simulink model "power_13NodeTestFeeder_4VSC_PV_DEG_symmtrc_loads_"  (R2024b)
settings: Solver=ode15s  StartTime=0.0  StopTime=5  FixedStep=1e-6  MaxStep=1e-4  RelTol=1e-6  AbsTol=1e-8  EnableMultiTasking=on
PreLoadFcn:
  | %power_13NodeTestFeeder_init;
values from neighbouring files (symbols this model uses):
  a = 1.3    [init_para_with_symmtrc_loads.m]
  Cdc = 278e-3    (= 0.278)    [init_para_with_symmtrc_loads.m]
  fg = 60    [a01_scan_VSC_13_feeder.m]    (also in init_para_with_symmtrc_loads.m)
  Gn = 1000    [init_para_with_symmtrc_loads.m]
  H = 8    [init_para_with_symmtrc_loads.m]
  Ipv_n = Isc_n*(Rp+Rs)/Rp    (= 8.21426513558)    [init_para_with_symmtrc_loads.m]
  Isc_n = 8.21    [init_para_with_symmtrc_loads.m]
  k = 1.3806503e-23    [init_para_with_symmtrc_loads.m]    (also in ypm_plot_compare_ana_meas.m = 2)
  Kdroop = Sn/(Rdroop*60)    (= 4166666.66667)    [init_para_with_symmtrc_loads.m]
  KI = 0.0032    [init_para_with_symmtrc_loads.m]
  Ki_C = Rc/tau_C    (= 0.768)    [init_para_with_symmtrc_loads.m]
  Ki_DC = omega_DC^2*Cdc    [init_para_with_symmtrc_loads.m]
  ki_dvpp = kp_dvpp/Ti_dvpp    [init_para_with_symmtrc_loads.m]
  Ki_P = 1/(Ki_pq*tau_P)    [init_para_with_symmtrc_loads.m]
  Ki_PLL = Kp_PLL/tau_PLL    [init_para_with_symmtrc_loads.m]
  Kp_C = Lc/tau_C    (= 0.020372)    [init_para_with_symmtrc_loads.m]
  Kp_DC = 2*xi_DC*omega_DC*Cdc    [init_para_with_symmtrc_loads.m]
  kp_dvpp = -(2*Kdcgain)^-1    [init_para_with_symmtrc_loads.m]
  Kp_P = tau_C/(Ki_pq*tau_P)    [init_para_with_symmtrc_loads.m]
  Kp_PLL = xi_PLL*2*omega_PLL/Vp    [init_para_with_symmtrc_loads.m]
  KV = -0.123    [init_para_with_symmtrc_loads.m]
  kv_Vp = [ 1.021 1.042 1.0174]    [init_para_with_symmtrc_loads.m]
  KVmp = Vmp_n/Voc_n    (= 0.799392097264)    [init_para_with_symmtrc_loads.m]
  Lc = 20.372e-6    (= 2.0372e-05)    [init_para_with_symmtrc_loads.m]
  Lg = Xg /(2*pi*fg)    [init_para_with_symmtrc_loads.m]
  Np = 345    [init_para_with_symmtrc_loads.m]
  Ns = 45    [init_para_with_symmtrc_loads.m]
  Ns_cell = 54    [init_para_with_symmtrc_loads.m]
  p_jump_time = 5    [init_para_with_symmtrc_loads.m]
  p_jump_value = 2*-1e6    (= -2000000)    [init_para_with_symmtrc_loads.m]
  phi_vec = phi_vec_deg/180*pi    [init_para_with_symmtrc_loads.m]
  ppv_nom = 4.9687e+05    (= 496870)    [init_para_with_symmtrc_loads.m]
  q = 1.6021764e-19    [init_para_with_symmtrc_loads.m]
  Rc = 0.768e-3    (= 0.000768)    [init_para_with_symmtrc_loads.m]
  Rg = (U_rms^2 / S_sc) / (sqrt(1 + XoverR^2))    [init_para_with_symmtrc_loads.m]
  Rp = 425.405    [init_para_with_symmtrc_loads.m]
  Rs = 0.221    [init_para_with_symmtrc_loads.m]
  S_base_all = 1    [init_para_with_symmtrc_loads.m]
  Sn = 15e6    (= 15000000)    [init_para_with_symmtrc_loads.m]
  tau_PLL = 2*xi_PLL/omega_PLL    [init_para_with_symmtrc_loads.m]
  Tn = 25    [init_para_with_symmtrc_loads.m]
  Ts = T_ctrl/n_ctrl    [a01_scan_VSC_13_feeder.m]    (also in init_para_with_symmtrc_loads.m = 5e-05)
  U_rms = 4160    [init_para_with_symmtrc_loads.m]
  Vdc = 1200    [init_para_with_symmtrc_loads.m]
  Voc_n = 32.9    [init_para_with_symmtrc_loads.m]
  Vp = sqrt(2)*480/sqrt(3)    [a01_scan_VSC_13_feeder.m]    (also in init_para_with_symmtrc_loads.m = Ug*sqrt(2)/sqrt(3))
undefined symbols (not defined in the file or in its folder): j, Newton, para_grid, para_PVgeno, Raphson
libraries: spsabctoAlphaBetaZeroLib x141, spsPower3phInstantaneousLib x70, spsSeriesRLCBranchLib x44, spsThreePhaseVIMeasurementLib x27, slpidlib x24, spsThreePhaseSeriesRLCLoadLib x15, spsControlledVoltageSourceLib x15, spsMeanLib x9, spsCurrentMeasurementLib x8, spsControlledCurrentSourceLib x8, cstblocks x8, spsGroundLib x5
(part 6 of 10)

== system power_13NodeTestFeeder_4VSC_PV_DEG_symmtrc_loads_/V I P Q Measurements EMT_without scopes_with_logsout/PQ_12 ==
  U : Inport
  I : Inport  Port=2
  Complex to Magnitude-Angle1 : ComplexToMagnitudeAngle
  Complex to Magnitude-Angle2 : ComplexToMagnitudeAngle
  Complex to Real-Imag : ComplexToRealImag
  Demux : Demux  Outputs=3
  Demux1 : Demux  Outputs=3
  Gain : Gain  Gain=1/S_base_all
  Gain1 : Gain  Gain=j
  Mux : Mux  Inputs=2
  "Power (3ph, Instantaneous)1" : spsPower3phInstantaneousLib/Power (3ph, Instantaneous)
  Real-Imag to Complex : RealImagToComplex
  Real-Imag to Complex1 : RealImagToComplex
  Sum : Sum  Inputs=|++
  Terminator{1,3,5..8} (6 alike) : Terminator
  Transfer Fcn{1..4} (4 alike) : TransferFcn  Denominator=[1e-3 1]
  abc to Alpha-Beta-Zero : spsabctoAlphaBetaZeroLib/abc to Alpha-Beta-Zero
  abc to Alpha-Beta-Zero1 : spsabctoAlphaBetaZeroLib/abc to Alpha-Beta-Zero
  PQ : Outport
  wires:
  I/1 -> abc to Alpha-Beta-Zero1/1, "Power (3ph, Instantaneous)1"/2
  Gain1/1 -> Sum/2
  Complex to Real-Imag/1 -> Mux/1
  Complex to Real-Imag/2 -> Mux/2
  Mux/1 -> PQ/1
  "Power (3ph, Instantaneous)1"/2 -> Transfer Fcn2/1
  "Power (3ph, Instantaneous)1"/1 -> Transfer Fcn1/1
  Sum/1 -> Gain/1
  Gain/1 -> Complex to Real-Imag/1
  U/1 -> abc to Alpha-Beta-Zero/1, "Power (3ph, Instantaneous)1"/1
  abc to Alpha-Beta-Zero/1 -> Demux/1
  Demux/1 -> Real-Imag to Complex/1
  Demux/2 -> Real-Imag to Complex/2
  Real-Imag to Complex/1 -> Complex to Magnitude-Angle2/1
  Complex to Magnitude-Angle2/1 -> Transfer Fcn3/1
  Complex to Magnitude-Angle2/2 -> Terminator3/1
  Complex to Magnitude-Angle1/1 -> Transfer Fcn4/1
  Real-Imag to Complex1/1 -> Complex to Magnitude-Angle1/1
  Demux1/2 -> Real-Imag to Complex1/2
  Demux1/1 -> Real-Imag to Complex1/1
  abc to Alpha-Beta-Zero1/1 -> Demux1/1
  Transfer Fcn1/1 -> Sum/1  "p"
  Transfer Fcn2/1 -> Gain1/1  "p"
  Transfer Fcn3/1 -> Terminator6/1  "u_betrag"
  Transfer Fcn4/1 -> Terminator5/1  "i_betrag"
  Demux1/3 -> Terminator7/1
  Demux/3 -> Terminator8/1
  Complex to Magnitude-Angle1/2 -> Terminator1/1

== system power_13NodeTestFeeder_4VSC_PV_DEG_symmtrc_loads_/V I P Q Measurements EMT_without scopes_with_logsout/PQ_13 ==
  U : Inport
  I : Inport  Port=2
  Complex to Magnitude-Angle1 : ComplexToMagnitudeAngle
  Complex to Magnitude-Angle2 : ComplexToMagnitudeAngle
  Complex to Real-Imag : ComplexToRealImag
  Demux : Demux  Outputs=3
  Demux1 : Demux  Outputs=3
  Gain : Gain  Gain=1/S_base_all
  Gain1 : Gain  Gain=j
  Mux : Mux  Inputs=2
  "Power (3ph, Instantaneous)1" : spsPower3phInstantaneousLib/Power (3ph, Instantaneous)
  Real-Imag to Complex : RealImagToComplex
  Real-Imag to Complex1 : RealImagToComplex
  Sum : Sum  Inputs=|++
  Terminator{1,3,5..8} (6 alike) : Terminator
  Transfer Fcn{1..4} (4 alike) : TransferFcn  Denominator=[1e-3 1]
  abc to Alpha-Beta-Zero : spsabctoAlphaBetaZeroLib/abc to Alpha-Beta-Zero
  abc to Alpha-Beta-Zero1 : spsabctoAlphaBetaZeroLib/abc to Alpha-Beta-Zero
  PQ : Outport
  wires:
  I/1 -> abc to Alpha-Beta-Zero1/1, "Power (3ph, Instantaneous)1"/2
  Gain1/1 -> Sum/2
  Complex to Real-Imag/1 -> Mux/1
  Complex to Real-Imag/2 -> Mux/2
  Mux/1 -> PQ/1
  "Power (3ph, Instantaneous)1"/2 -> Transfer Fcn2/1
  "Power (3ph, Instantaneous)1"/1 -> Transfer Fcn1/1
  Sum/1 -> Gain/1
  Gain/1 -> Complex to Real-Imag/1
  U/1 -> abc to Alpha-Beta-Zero/1, "Power (3ph, Instantaneous)1"/1
  abc to Alpha-Beta-Zero/1 -> Demux/1
  Demux/1 -> Real-Imag to Complex/1
  Demux/2 -> Real-Imag to Complex/2
  Real-Imag to Complex/1 -> Complex to Magnitude-Angle2/1
  Complex to Magnitude-Angle2/1 -> Transfer Fcn3/1
  Complex to Magnitude-Angle2/2 -> Terminator3/1
  Complex to Magnitude-Angle1/1 -> Transfer Fcn4/1
  Real-Imag to Complex1/1 -> Complex to Magnitude-Angle1/1
  Demux1/2 -> Real-Imag to Complex1/2
  Demux1/1 -> Real-Imag to Complex1/1
  abc to Alpha-Beta-Zero1/1 -> Demux1/1
  Transfer Fcn1/1 -> Sum/1  "p"
  Transfer Fcn2/1 -> Gain1/1  "p"
  Transfer Fcn3/1 -> Terminator6/1  "u_betrag"
  Transfer Fcn4/1 -> Terminator5/1  "i_betrag"
  Demux1/3 -> Terminator7/1
  Demux/3 -> Terminator8/1
  Complex to Magnitude-Angle1/2 -> Terminator1/1

== system power_13NodeTestFeeder_4VSC_PV_DEG_symmtrc_loads_/V I P Q Measurements EMT_without scopes_with_logsout/PQ_14 ==
  U : Inport
  I : Inport  Port=2
  Complex to Magnitude-Angle1 : ComplexToMagnitudeAngle
  Complex to Magnitude-Angle2 : ComplexToMagnitudeAngle
  Complex to Real-Imag : ComplexToRealImag
  Demux : Demux  Outputs=3
  Demux1 : Demux  Outputs=3
  Gain : Gain  Gain=1/S_base_all
  Gain1 : Gain  Gain=j
  Mux : Mux  Inputs=2
  "Power (3ph, Instantaneous)1" : spsPower3phInstantaneousLib/Power (3ph, Instantaneous)
  Real-Imag to Complex : RealImagToComplex
  Real-Imag to Complex1 : RealImagToComplex
  Sum : Sum  Inputs=|++
  Terminator{1,3,5..8} (6 alike) : Terminator
  Transfer Fcn{1..4} (4 alike) : TransferFcn  Denominator=[1e-3 1]
  abc to Alpha-Beta-Zero : spsabctoAlphaBetaZeroLib/abc to Alpha-Beta-Zero
  abc to Alpha-Beta-Zero1 : spsabctoAlphaBetaZeroLib/abc to Alpha-Beta-Zero
  PQ : Outport
  wires:
  I/1 -> abc to Alpha-Beta-Zero1/1, "Power (3ph, Instantaneous)1"/2
  Gain1/1 -> Sum/2
  Complex to Real-Imag/1 -> Mux/1
  Complex to Real-Imag/2 -> Mux/2
  Mux/1 -> PQ/1
  "Power (3ph, Instantaneous)1"/2 -> Transfer Fcn2/1
  "Power (3ph, Instantaneous)1"/1 -> Transfer Fcn1/1
  Sum/1 -> Gain/1
  Gain/1 -> Complex to Real-Imag/1
  U/1 -> abc to Alpha-Beta-Zero/1, "Power (3ph, Instantaneous)1"/1
  abc to Alpha-Beta-Zero/1 -> Demux/1
  Demux/1 -> Real-Imag to Complex/1
  Demux/2 -> Real-Imag to Complex/2
  Real-Imag to Complex/1 -> Complex to Magnitude-Angle2/1
  Complex to Magnitude-Angle2/1 -> Transfer Fcn3/1
  Complex to Magnitude-Angle2/2 -> Terminator3/1
  Complex to Magnitude-Angle1/1 -> Transfer Fcn4/1
  Real-Imag to Complex1/1 -> Complex to Magnitude-Angle1/1
  Demux1/2 -> Real-Imag to Complex1/2
  Demux1/1 -> Real-Imag to Complex1/1
  abc to Alpha-Beta-Zero1/1 -> Demux1/1
  Transfer Fcn1/1 -> Sum/1  "p"
  Transfer Fcn2/1 -> Gain1/1  "p"
  Transfer Fcn3/1 -> Terminator6/1  "u_betrag"
  Transfer Fcn4/1 -> Terminator5/1  "i_betrag"
  Demux1/3 -> Terminator7/1
  Demux/3 -> Terminator8/1
  Complex to Magnitude-Angle1/2 -> Terminator1/1

== system power_13NodeTestFeeder_4VSC_PV_DEG_symmtrc_loads_/V I P Q Measurements EMT_without scopes_with_logsout/PQ_15 ==
  U : Inport
  I : Inport  Port=2
  Complex to Magnitude-Angle1 : ComplexToMagnitudeAngle
  Complex to Magnitude-Angle2 : ComplexToMagnitudeAngle
  Complex to Real-Imag : ComplexToRealImag
  Demux : Demux  Outputs=3
  Demux1 : Demux  Outputs=3
  Gain : Gain  Gain=1/S_base_all
  Gain1 : Gain  Gain=j
  Mux : Mux  Inputs=2
  "Power (3ph, Instantaneous)1" : spsPower3phInstantaneousLib/Power (3ph, Instantaneous)
  Real-Imag to Complex : RealImagToComplex
  Real-Imag to Complex1 : RealImagToComplex
  Sum : Sum  Inputs=|++
  Terminator{1,3,5..8} (6 alike) : Terminator
  Transfer Fcn{1..4} (4 alike) : TransferFcn  Denominator=[1e-3 1]
  abc to Alpha-Beta-Zero : spsabctoAlphaBetaZeroLib/abc to Alpha-Beta-Zero
  abc to Alpha-Beta-Zero1 : spsabctoAlphaBetaZeroLib/abc to Alpha-Beta-Zero
  PQ : Outport
  wires:
  I/1 -> abc to Alpha-Beta-Zero1/1, "Power (3ph, Instantaneous)1"/2
  Gain1/1 -> Sum/2
  Complex to Real-Imag/1 -> Mux/1
  Complex to Real-Imag/2 -> Mux/2
  Mux/1 -> PQ/1
  "Power (3ph, Instantaneous)1"/2 -> Transfer Fcn2/1
  "Power (3ph, Instantaneous)1"/1 -> Transfer Fcn1/1
  Sum/1 -> Gain/1
  Gain/1 -> Complex to Real-Imag/1
  U/1 -> abc to Alpha-Beta-Zero/1, "Power (3ph, Instantaneous)1"/1
  abc to Alpha-Beta-Zero/1 -> Demux/1
  Demux/1 -> Real-Imag to Complex/1
  Demux/2 -> Real-Imag to Complex/2
  Real-Imag to Complex/1 -> Complex to Magnitude-Angle2/1
  Complex to Magnitude-Angle2/1 -> Transfer Fcn3/1
  Complex to Magnitude-Angle2/2 -> Terminator3/1
  Complex to Magnitude-Angle1/1 -> Transfer Fcn4/1
  Real-Imag to Complex1/1 -> Complex to Magnitude-Angle1/1
  Demux1/2 -> Real-Imag to Complex1/2
  Demux1/1 -> Real-Imag to Complex1/1
  abc to Alpha-Beta-Zero1/1 -> Demux1/1
  Transfer Fcn1/1 -> Sum/1  "p"
  Transfer Fcn2/1 -> Gain1/1  "p"
  Transfer Fcn3/1 -> Terminator6/1  "u_betrag"
  Transfer Fcn4/1 -> Terminator5/1  "i_betrag"
  Demux1/3 -> Terminator7/1
  Demux/3 -> Terminator8/1
  Complex to Magnitude-Angle1/2 -> Terminator1/1

== system power_13NodeTestFeeder_4VSC_PV_DEG_symmtrc_loads_/V I P Q Measurements EMT_without scopes_with_logsout/PQ_16 ==
  U : Inport
  I : Inport  Port=2
  Complex to Magnitude-Angle1 : ComplexToMagnitudeAngle
  Complex to Magnitude-Angle2 : ComplexToMagnitudeAngle
  Complex to Real-Imag : ComplexToRealImag
  Demux : Demux  Outputs=3
  Demux1 : Demux  Outputs=3
  Gain : Gain  Gain=1/S_base_all
  Gain1 : Gain  Gain=j
  Mux : Mux  Inputs=2
  "Power (3ph, Instantaneous)1" : spsPower3phInstantaneousLib/Power (3ph, Instantaneous)
  Real-Imag to Complex : RealImagToComplex
  Real-Imag to Complex1 : RealImagToComplex
  Sum : Sum  Inputs=|++
  Terminator{1,3,5..8} (6 alike) : Terminator
  Transfer Fcn{1..4} (4 alike) : TransferFcn  Denominator=[1e-3 1]
  abc to Alpha-Beta-Zero : spsabctoAlphaBetaZeroLib/abc to Alpha-Beta-Zero
  abc to Alpha-Beta-Zero1 : spsabctoAlphaBetaZeroLib/abc to Alpha-Beta-Zero
  PQ : Outport
  wires:
  I/1 -> abc to Alpha-Beta-Zero1/1, "Power (3ph, Instantaneous)1"/2
  Gain1/1 -> Sum/2
  Complex to Real-Imag/1 -> Mux/1
  Complex to Real-Imag/2 -> Mux/2
  Mux/1 -> PQ/1
  "Power (3ph, Instantaneous)1"/2 -> Transfer Fcn2/1
  "Power (3ph, Instantaneous)1"/1 -> Transfer Fcn1/1
  Sum/1 -> Gain/1
  Gain/1 -> Complex to Real-Imag/1
  U/1 -> abc to Alpha-Beta-Zero/1, "Power (3ph, Instantaneous)1"/1
  abc to Alpha-Beta-Zero/1 -> Demux/1
  Demux/1 -> Real-Imag to Complex/1
  Demux/2 -> Real-Imag to Complex/2
  Real-Imag to Complex/1 -> Complex to Magnitude-Angle2/1
  Complex to Magnitude-Angle2/1 -> Transfer Fcn3/1
  Complex to Magnitude-Angle2/2 -> Terminator3/1
  Complex to Magnitude-Angle1/1 -> Transfer Fcn4/1
  Real-Imag to Complex1/1 -> Complex to Magnitude-Angle1/1
  Demux1/2 -> Real-Imag to Complex1/2
  Demux1/1 -> Real-Imag to Complex1/1
  abc to Alpha-Beta-Zero1/1 -> Demux1/1
  Transfer Fcn1/1 -> Sum/1  "p"
  Transfer Fcn2/1 -> Gain1/1  "p"
  Transfer Fcn3/1 -> Terminator6/1  "u_betrag"
  Transfer Fcn4/1 -> Terminator5/1  "i_betrag"
  Demux1/3 -> Terminator7/1
  Demux/3 -> Terminator8/1
  Complex to Magnitude-Angle1/2 -> Terminator1/1

== system power_13NodeTestFeeder_4VSC_PV_DEG_symmtrc_loads_/V I P Q Measurements EMT_without scopes_with_logsout/PQ_17 ==
  U : Inport
  I : Inport  Port=2
  Complex to Magnitude-Angle1 : ComplexToMagnitudeAngle
  Complex to Magnitude-Angle2 : ComplexToMagnitudeAngle
  Complex to Real-Imag : ComplexToRealImag
  Demux : Demux  Outputs=3
  Demux1 : Demux  Outputs=3
  Gain : Gain  Gain=1/S_base_all
  Gain1 : Gain  Gain=j
  Mux : Mux  Inputs=2
  "Power (3ph, Instantaneous)1" : spsPower3phInstantaneousLib/Power (3ph, Instantaneous)
  Real-Imag to Complex : RealImagToComplex
  Real-Imag to Complex1 : RealImagToComplex
  Sum : Sum  Inputs=|++
  Terminator{1,3,5..8} (6 alike) : Terminator
  Transfer Fcn{1..4} (4 alike) : TransferFcn  Denominator=[1e-3 1]
  abc to Alpha-Beta-Zero : spsabctoAlphaBetaZeroLib/abc to Alpha-Beta-Zero
  abc to Alpha-Beta-Zero1 : spsabctoAlphaBetaZeroLib/abc to Alpha-Beta-Zero
  PQ : Outport
  wires:
  I/1 -> abc to Alpha-Beta-Zero1/1, "Power (3ph, Instantaneous)1"/2
  Gain1/1 -> Sum/2
  Complex to Real-Imag/1 -> Mux/1
  Complex to Real-Imag/2 -> Mux/2
  Mux/1 -> PQ/1
  "Power (3ph, Instantaneous)1"/2 -> Transfer Fcn2/1
  "Power (3ph, Instantaneous)1"/1 -> Transfer Fcn1/1
  Sum/1 -> Gain/1
  Gain/1 -> Complex to Real-Imag/1
  U/1 -> abc to Alpha-Beta-Zero/1, "Power (3ph, Instantaneous)1"/1
  abc to Alpha-Beta-Zero/1 -> Demux/1
  Demux/1 -> Real-Imag to Complex/1
  Demux/2 -> Real-Imag to Complex/2
  Real-Imag to Complex/1 -> Complex to Magnitude-Angle2/1
  Complex to Magnitude-Angle2/1 -> Transfer Fcn3/1
  Complex to Magnitude-Angle2/2 -> Terminator3/1
  Complex to Magnitude-Angle1/1 -> Transfer Fcn4/1
  Real-Imag to Complex1/1 -> Complex to Magnitude-Angle1/1
  Demux1/2 -> Real-Imag to Complex1/2
  Demux1/1 -> Real-Imag to Complex1/1
  abc to Alpha-Beta-Zero1/1 -> Demux1/1
  Transfer Fcn1/1 -> Sum/1  "p"
  Transfer Fcn2/1 -> Gain1/1  "p"
  Transfer Fcn3/1 -> Terminator6/1  "u_betrag"
  Transfer Fcn4/1 -> Terminator5/1  "i_betrag"
  Demux1/3 -> Terminator7/1
  Demux/3 -> Terminator8/1
  Complex to Magnitude-Angle1/2 -> Terminator1/1

== system power_13NodeTestFeeder_4VSC_PV_DEG_symmtrc_loads_/V I P Q Measurements EMT_without scopes_with_logsout/PQ_18 ==
  U : Inport
  I : Inport  Port=2
  Complex to Magnitude-Angle1 : ComplexToMagnitudeAngle
  Complex to Magnitude-Angle2 : ComplexToMagnitudeAngle
  Complex to Real-Imag : ComplexToRealImag
  Demux : Demux  Outputs=3
  Demux1 : Demux  Outputs=3
  Gain : Gain  Gain=1/S_base_all
  Gain1 : Gain  Gain=j
  Mux : Mux  Inputs=2
  "Power (3ph, Instantaneous)1" : spsPower3phInstantaneousLib/Power (3ph, Instantaneous)
  Real-Imag to Complex : RealImagToComplex
  Real-Imag to Complex1 : RealImagToComplex
  Sum : Sum  Inputs=|++
  Terminator{1,3,5..8} (6 alike) : Terminator
  Transfer Fcn{1..4} (4 alike) : TransferFcn  Denominator=[1e-3 1]
  abc to Alpha-Beta-Zero : spsabctoAlphaBetaZeroLib/abc to Alpha-Beta-Zero
  abc to Alpha-Beta-Zero1 : spsabctoAlphaBetaZeroLib/abc to Alpha-Beta-Zero
  PQ : Outport
  wires:
  I/1 -> abc to Alpha-Beta-Zero1/1, "Power (3ph, Instantaneous)1"/2
  Gain1/1 -> Sum/2
  Complex to Real-Imag/1 -> Mux/1
  Complex to Real-Imag/2 -> Mux/2
  Mux/1 -> PQ/1
  "Power (3ph, Instantaneous)1"/2 -> Transfer Fcn2/1
  "Power (3ph, Instantaneous)1"/1 -> Transfer Fcn1/1
  Sum/1 -> Gain/1
  Gain/1 -> Complex to Real-Imag/1
  U/1 -> abc to Alpha-Beta-Zero/1, "Power (3ph, Instantaneous)1"/1
  abc to Alpha-Beta-Zero/1 -> Demux/1
  Demux/1 -> Real-Imag to Complex/1
  Demux/2 -> Real-Imag to Complex/2
  Real-Imag to Complex/1 -> Complex to Magnitude-Angle2/1
  Complex to Magnitude-Angle2/1 -> Transfer Fcn3/1
  Complex to Magnitude-Angle2/2 -> Terminator3/1
  Complex to Magnitude-Angle1/1 -> Transfer Fcn4/1
  Real-Imag to Complex1/1 -> Complex to Magnitude-Angle1/1
  Demux1/2 -> Real-Imag to Complex1/2
  Demux1/1 -> Real-Imag to Complex1/1
  abc to Alpha-Beta-Zero1/1 -> Demux1/1
  Transfer Fcn1/1 -> Sum/1  "p"
  Transfer Fcn2/1 -> Gain1/1  "p"
  Transfer Fcn3/1 -> Terminator6/1  "u_betrag"
  Transfer Fcn4/1 -> Terminator5/1  "i_betrag"
  Demux1/3 -> Terminator7/1
  Demux/3 -> Terminator8/1
  Complex to Magnitude-Angle1/2 -> Terminator1/1

== system power_13NodeTestFeeder_4VSC_PV_DEG_symmtrc_loads_/V I P Q Measurements EMT_without scopes_with_logsout/PQ_19 ==
  U : Inport
  I : Inport  Port=2
  Complex to Magnitude-Angle1 : ComplexToMagnitudeAngle
  Complex to Magnitude-Angle2 : ComplexToMagnitudeAngle
  Complex to Real-Imag : ComplexToRealImag
  Demux : Demux  Outputs=3
  Demux1 : Demux  Outputs=3
  Gain : Gain  Gain=1/S_base_all
  Gain1 : Gain  Gain=j
  Mux : Mux  Inputs=2
  "Power (3ph, Instantaneous)1" : spsPower3phInstantaneousLib/Power (3ph, Instantaneous)
  Real-Imag to Complex : RealImagToComplex
  Real-Imag to Complex1 : RealImagToComplex
  Sum : Sum  Inputs=|++
  Terminator{1,3,5..8} (6 alike) : Terminator
  Transfer Fcn{1..4} (4 alike) : TransferFcn  Denominator=[1e-3 1]
  abc to Alpha-Beta-Zero : spsabctoAlphaBetaZeroLib/abc to Alpha-Beta-Zero
  abc to Alpha-Beta-Zero1 : spsabctoAlphaBetaZeroLib/abc to Alpha-Beta-Zero
  PQ : Outport
  wires:
  I/1 -> abc to Alpha-Beta-Zero1/1, "Power (3ph, Instantaneous)1"/2
  Gain1/1 -> Sum/2
  Complex to Real-Imag/1 -> Mux/1
  Complex to Real-Imag/2 -> Mux/2
  Mux/1 -> PQ/1
  "Power (3ph, Instantaneous)1"/2 -> Transfer Fcn2/1
  "Power (3ph, Instantaneous)1"/1 -> Transfer Fcn1/1
  Sum/1 -> Gain/1
  Gain/1 -> Complex to Real-Imag/1
  U/1 -> abc to Alpha-Beta-Zero/1, "Power (3ph, Instantaneous)1"/1
  abc to Alpha-Beta-Zero/1 -> Demux/1
  Demux/1 -> Real-Imag to Complex/1
  Demux/2 -> Real-Imag to Complex/2
  Real-Imag to Complex/1 -> Complex to Magnitude-Angle2/1
  Complex to Magnitude-Angle2/1 -> Transfer Fcn3/1
  Complex to Magnitude-Angle2/2 -> Terminator3/1
  Complex to Magnitude-Angle1/1 -> Transfer Fcn4/1
  Real-Imag to Complex1/1 -> Complex to Magnitude-Angle1/1
  Demux1/2 -> Real-Imag to Complex1/2
  Demux1/1 -> Real-Imag to Complex1/1
  abc to Alpha-Beta-Zero1/1 -> Demux1/1
  Transfer Fcn1/1 -> Sum/1  "p"
  Transfer Fcn2/1 -> Gain1/1  "p"
  Transfer Fcn3/1 -> Terminator6/1  "u_betrag"
  Transfer Fcn4/1 -> Terminator5/1  "i_betrag"
  Demux1/3 -> Terminator7/1
  Demux/3 -> Terminator8/1
  Complex to Magnitude-Angle1/2 -> Terminator1/1

== system power_13NodeTestFeeder_4VSC_PV_DEG_symmtrc_loads_/V I P Q Measurements EMT_without scopes_with_logsout/PQ_2 ==
  U : Inport
  I : Inport  Port=2
  Complex to Magnitude-Angle1 : ComplexToMagnitudeAngle
  Complex to Magnitude-Angle2 : ComplexToMagnitudeAngle
  Complex to Real-Imag : ComplexToRealImag
  Demux : Demux  Outputs=3
  Demux1 : Demux  Outputs=3
  Gain : Gain  Gain=1/S_base_all
  Gain1 : Gain  Gain=j
  Mux : Mux  Inputs=2
  "Power (3ph, Instantaneous)1" : spsPower3phInstantaneousLib/Power (3ph, Instantaneous)
  Real-Imag to Complex : RealImagToComplex
  Real-Imag to Complex1 : RealImagToComplex
  Sum : Sum  Inputs=|++
  Terminator{1,3,5..8} (6 alike) : Terminator
  Transfer Fcn{1..4} (4 alike) : TransferFcn  Denominator=[1e-3 1]
  abc to Alpha-Beta-Zero : spsabctoAlphaBetaZeroLib/abc to Alpha-Beta-Zero
  abc to Alpha-Beta-Zero1 : spsabctoAlphaBetaZeroLib/abc to Alpha-Beta-Zero
  PQ : Outport
  wires:
  I/1 -> abc to Alpha-Beta-Zero1/1, "Power (3ph, Instantaneous)1"/2
  Gain1/1 -> Sum/2
  Complex to Real-Imag/1 -> Mux/1
  Complex to Real-Imag/2 -> Mux/2
  Mux/1 -> PQ/1
  "Power (3ph, Instantaneous)1"/2 -> Transfer Fcn2/1
  "Power (3ph, Instantaneous)1"/1 -> Transfer Fcn1/1
  Sum/1 -> Gain/1
  Gain/1 -> Complex to Real-Imag/1
  U/1 -> abc to Alpha-Beta-Zero/1, "Power (3ph, Instantaneous)1"/1
  abc to Alpha-Beta-Zero/1 -> Demux/1
  Demux/1 -> Real-Imag to Complex/1
  Demux/2 -> Real-Imag to Complex/2
  Real-Imag to Complex/1 -> Complex to Magnitude-Angle2/1
  Complex to Magnitude-Angle2/1 -> Transfer Fcn3/1
  Complex to Magnitude-Angle2/2 -> Terminator3/1
  Complex to Magnitude-Angle1/1 -> Transfer Fcn4/1
  Real-Imag to Complex1/1 -> Complex to Magnitude-Angle1/1
  Demux1/2 -> Real-Imag to Complex1/2
  Demux1/1 -> Real-Imag to Complex1/1
  abc to Alpha-Beta-Zero1/1 -> Demux1/1
  Transfer Fcn1/1 -> Sum/1  "p"
  Transfer Fcn2/1 -> Gain1/1  "p"
  Transfer Fcn3/1 -> Terminator6/1  "u_betrag"
  Transfer Fcn4/1 -> Terminator5/1  "i_betrag"
  Demux1/3 -> Terminator7/1
  Demux/3 -> Terminator8/1
  Complex to Magnitude-Angle1/2 -> Terminator1/1

== system power_13NodeTestFeeder_4VSC_PV_DEG_symmtrc_loads_/V I P Q Measurements EMT_without scopes_with_logsout/PQ_3 ==
  U : Inport
  I : Inport  Port=2
  Complex to Magnitude-Angle1 : ComplexToMagnitudeAngle
  Complex to Magnitude-Angle2 : ComplexToMagnitudeAngle
  Complex to Real-Imag : ComplexToRealImag
  Demux : Demux  Outputs=3
  Demux1 : Demux  Outputs=3
  Gain : Gain  Gain=1/S_base_all
  Gain1 : Gain  Gain=j
  Mux : Mux  Inputs=2
  "Power (3ph, Instantaneous)1" : spsPower3phInstantaneousLib/Power (3ph, Instantaneous)
  Real-Imag to Complex : RealImagToComplex
  Real-Imag to Complex1 : RealImagToComplex
  Sum : Sum  Inputs=|++
  Terminator{1,3,5..8} (6 alike) : Terminator
  Transfer Fcn{1..4} (4 alike) : TransferFcn  Denominator=[1e-3 1]
  abc to Alpha-Beta-Zero : spsabctoAlphaBetaZeroLib/abc to Alpha-Beta-Zero
  abc to Alpha-Beta-Zero1 : spsabctoAlphaBetaZeroLib/abc to Alpha-Beta-Zero
  PQ : Outport
  wires:
  I/1 -> abc to Alpha-Beta-Zero1/1, "Power (3ph, Instantaneous)1"/2
  Gain1/1 -> Sum/2
  Complex to Real-Imag/1 -> Mux/1
  Complex to Real-Imag/2 -> Mux/2
  Mux/1 -> PQ/1
  "Power (3ph, Instantaneous)1"/2 -> Transfer Fcn2/1
  "Power (3ph, Instantaneous)1"/1 -> Transfer Fcn1/1
  Sum/1 -> Gain/1
  Gain/1 -> Complex to Real-Imag/1
  U/1 -> abc to Alpha-Beta-Zero/1, "Power (3ph, Instantaneous)1"/1
  abc to Alpha-Beta-Zero/1 -> Demux/1
  Demux/1 -> Real-Imag to Complex/1
  Demux/2 -> Real-Imag to Complex/2
  Real-Imag to Complex/1 -> Complex to Magnitude-Angle2/1
  Complex to Magnitude-Angle2/1 -> Transfer Fcn3/1
  Complex to Magnitude-Angle2/2 -> Terminator3/1
  Complex to Magnitude-Angle1/1 -> Transfer Fcn4/1
  Real-Imag to Complex1/1 -> Complex to Magnitude-Angle1/1
  Demux1/2 -> Real-Imag to Complex1/2
  Demux1/1 -> Real-Imag to Complex1/1
  abc to Alpha-Beta-Zero1/1 -> Demux1/1
  Transfer Fcn1/1 -> Sum/1  "p"
  Transfer Fcn2/1 -> Gain1/1  "p"
  Transfer Fcn3/1 -> Terminator6/1  "u_betrag"
  Transfer Fcn4/1 -> Terminator5/1  "i_betrag"
  Demux1/3 -> Terminator7/1
  Demux/3 -> Terminator8/1
  Complex to Magnitude-Angle1/2 -> Terminator1/1

== system power_13NodeTestFeeder_4VSC_PV_DEG_symmtrc_loads_/V I P Q Measurements EMT_without scopes_with_logsout/PQ_4 ==
  U : Inport
  I : Inport  Port=2
  Complex to Magnitude-Angle1 : ComplexToMagnitudeAngle
  Complex to Magnitude-Angle2 : ComplexToMagnitudeAngle
  Complex to Real-Imag : ComplexToRealImag
  Demux : Demux  Outputs=3
  Demux1 : Demux  Outputs=3
  Gain : Gain  Gain=1/S_base_all
  Gain1 : Gain  Gain=j
  Mux : Mux  Inputs=2
  "Power (3ph, Instantaneous)1" : spsPower3phInstantaneousLib/Power (3ph, Instantaneous)
  Real-Imag to Complex : RealImagToComplex
  Real-Imag to Complex1 : RealImagToComplex
  Sum : Sum  Inputs=|++
  Terminator{1,3,5..8} (6 alike) : Terminator
  Transfer Fcn{1..4} (4 alike) : TransferFcn  Denominator=[1e-3 1]
  abc to Alpha-Beta-Zero : spsabctoAlphaBetaZeroLib/abc to Alpha-Beta-Zero
  abc to Alpha-Beta-Zero1 : spsabctoAlphaBetaZeroLib/abc to Alpha-Beta-Zero
  PQ : Outport
  wires:
  I/1 -> abc to Alpha-Beta-Zero1/1, "Power (3ph, Instantaneous)1"/2
  Gain1/1 -> Sum/2
  Complex to Real-Imag/1 -> Mux/1
  Complex to Real-Imag/2 -> Mux/2
  Mux/1 -> PQ/1
  "Power (3ph, Instantaneous)1"/2 -> Transfer Fcn2/1
  "Power (3ph, Instantaneous)1"/1 -> Transfer Fcn1/1
  Sum/1 -> Gain/1
  Gain/1 -> Complex to Real-Imag/1
  U/1 -> abc to Alpha-Beta-Zero/1, "Power (3ph, Instantaneous)1"/1
  abc to Alpha-Beta-Zero/1 -> Demux/1
  Demux/1 -> Real-Imag to Complex/1
  Demux/2 -> Real-Imag to Complex/2
  Real-Imag to Complex/1 -> Complex to Magnitude-Angle2/1
  Complex to Magnitude-Angle2/1 -> Transfer Fcn3/1
  Complex to Magnitude-Angle2/2 -> Terminator3/1
  Complex to Magnitude-Angle1/1 -> Transfer Fcn4/1
  Real-Imag to Complex1/1 -> Complex to Magnitude-Angle1/1
  Demux1/2 -> Real-Imag to Complex1/2
  Demux1/1 -> Real-Imag to Complex1/1
  abc to Alpha-Beta-Zero1/1 -> Demux1/1
  Transfer Fcn1/1 -> Sum/1  "p"
  Transfer Fcn2/1 -> Gain1/1  "p"
  Transfer Fcn3/1 -> Terminator6/1  "u_betrag"
  Transfer Fcn4/1 -> Terminator5/1  "i_betrag"
  Demux1/3 -> Terminator7/1
  Demux/3 -> Terminator8/1
  Complex to Magnitude-Angle1/2 -> Terminator1/1

== system power_13NodeTestFeeder_4VSC_PV_DEG_symmtrc_loads_/V I P Q Measurements EMT_without scopes_with_logsout/PQ_5 ==
  U : Inport
  I : Inport  Port=2
  Complex to Magnitude-Angle1 : ComplexToMagnitudeAngle
  Complex to Magnitude-Angle2 : ComplexToMagnitudeAngle
  Complex to Real-Imag : ComplexToRealImag
  Demux : Demux  Outputs=3
  Demux1 : Demux  Outputs=3
  Gain : Gain  Gain=1/S_base_all
  Gain1 : Gain  Gain=j
  Mux : Mux  Inputs=2
  "Power (3ph, Instantaneous)1" : spsPower3phInstantaneousLib/Power (3ph, Instantaneous)
  Real-Imag to Complex : RealImagToComplex
  Real-Imag to Complex1 : RealImagToComplex
  Sum : Sum  Inputs=|++
  Terminator{1,3,5..8} (6 alike) : Terminator
  Transfer Fcn{1..4} (4 alike) : TransferFcn  Denominator=[1e-3 1]
  abc to Alpha-Beta-Zero : spsabctoAlphaBetaZeroLib/abc to Alpha-Beta-Zero
  abc to Alpha-Beta-Zero1 : spsabctoAlphaBetaZeroLib/abc to Alpha-Beta-Zero
  PQ : Outport
  wires:
  I/1 -> abc to Alpha-Beta-Zero1/1, "Power (3ph, Instantaneous)1"/2
  Gain1/1 -> Sum/2
  Complex to Real-Imag/1 -> Mux/1
  Complex to Real-Imag/2 -> Mux/2
  Mux/1 -> PQ/1
  "Power (3ph, Instantaneous)1"/2 -> Transfer Fcn2/1
  "Power (3ph, Instantaneous)1"/1 -> Transfer Fcn1/1
  Sum/1 -> Gain/1
  Gain/1 -> Complex to Real-Imag/1
  U/1 -> abc to Alpha-Beta-Zero/1, "Power (3ph, Instantaneous)1"/1
  abc to Alpha-Beta-Zero/1 -> Demux/1
  Demux/1 -> Real-Imag to Complex/1
  Demux/2 -> Real-Imag to Complex/2
  Real-Imag to Complex/1 -> Complex to Magnitude-Angle2/1
  Complex to Magnitude-Angle2/1 -> Transfer Fcn3/1
  Complex to Magnitude-Angle2/2 -> Terminator3/1
  Complex to Magnitude-Angle1/1 -> Transfer Fcn4/1
  Real-Imag to Complex1/1 -> Complex to Magnitude-Angle1/1
  Demux1/2 -> Real-Imag to Complex1/2
  Demux1/1 -> Real-Imag to Complex1/1
  abc to Alpha-Beta-Zero1/1 -> Demux1/1
  Transfer Fcn1/1 -> Sum/1  "p"
  Transfer Fcn2/1 -> Gain1/1  "p"
  Transfer Fcn3/1 -> Terminator6/1  "u_betrag"
  Transfer Fcn4/1 -> Terminator5/1  "i_betrag"
  Demux1/3 -> Terminator7/1
  Demux/3 -> Terminator8/1
  Complex to Magnitude-Angle1/2 -> Terminator1/1

== system power_13NodeTestFeeder_4VSC_PV_DEG_symmtrc_loads_/V I P Q Measurements EMT_without scopes_with_logsout/PQ_6 ==
  U : Inport
  I : Inport  Port=2
  Complex to Magnitude-Angle1 : ComplexToMagnitudeAngle
  Complex to Magnitude-Angle2 : ComplexToMagnitudeAngle
  Complex to Real-Imag : ComplexToRealImag
  Demux : Demux  Outputs=3
  Demux1 : Demux  Outputs=3
  Gain : Gain  Gain=1/S_base_all
  Gain1 : Gain  Gain=j
  Mux : Mux  Inputs=2
  "Power (3ph, Instantaneous)1" : spsPower3phInstantaneousLib/Power (3ph, Instantaneous)
  Real-Imag to Complex : RealImagToComplex
  Real-Imag to Complex1 : RealImagToComplex
  Sum : Sum  Inputs=|++
  Terminator{1,3,5..8} (6 alike) : Terminator
  Transfer Fcn{1..4} (4 alike) : TransferFcn  Denominator=[1e-3 1]
  abc to Alpha-Beta-Zero : spsabctoAlphaBetaZeroLib/abc to Alpha-Beta-Zero
  abc to Alpha-Beta-Zero1 : spsabctoAlphaBetaZeroLib/abc to Alpha-Beta-Zero
  PQ : Outport
  wires:
  I/1 -> abc to Alpha-Beta-Zero1/1, "Power (3ph, Instantaneous)1"/2
  Gain1/1 -> Sum/2
  Complex to Real-Imag/1 -> Mux/1
  Complex to Real-Imag/2 -> Mux/2
  Mux/1 -> PQ/1
  "Power (3ph, Instantaneous)1"/2 -> Transfer Fcn2/1
  "Power (3ph, Instantaneous)1"/1 -> Transfer Fcn1/1
  Sum/1 -> Gain/1
  Gain/1 -> Complex to Real-Imag/1
  U/1 -> abc to Alpha-Beta-Zero/1, "Power (3ph, Instantaneous)1"/1
  abc to Alpha-Beta-Zero/1 -> Demux/1
  Demux/1 -> Real-Imag to Complex/1
  Demux/2 -> Real-Imag to Complex/2
  Real-Imag to Complex/1 -> Complex to Magnitude-Angle2/1
  Complex to Magnitude-Angle2/1 -> Transfer Fcn3/1
  Complex to Magnitude-Angle2/2 -> Terminator3/1
  Complex to Magnitude-Angle1/1 -> Transfer Fcn4/1
  Real-Imag to Complex1/1 -> Complex to Magnitude-Angle1/1
  Demux1/2 -> Real-Imag to Complex1/2
  Demux1/1 -> Real-Imag to Complex1/1
  abc to Alpha-Beta-Zero1/1 -> Demux1/1
  Transfer Fcn1/1 -> Sum/1  "p"
  Transfer Fcn2/1 -> Gain1/1  "p"
  Transfer Fcn3/1 -> Terminator6/1  "u_betrag"
  Transfer Fcn4/1 -> Terminator5/1  "i_betrag"
  Demux1/3 -> Terminator7/1
  Demux/3 -> Terminator8/1
  Complex to Magnitude-Angle1/2 -> Terminator1/1

== system power_13NodeTestFeeder_4VSC_PV_DEG_symmtrc_loads_/V I P Q Measurements EMT_without scopes_with_logsout/PQ_7 ==
  U : Inport
  I : Inport  Port=2
  Complex to Magnitude-Angle1 : ComplexToMagnitudeAngle
  Complex to Magnitude-Angle2 : ComplexToMagnitudeAngle
  Complex to Real-Imag : ComplexToRealImag
  Demux : Demux  Outputs=3
  Demux1 : Demux  Outputs=3
  Gain : Gain  Gain=1/S_base_all
  Gain1 : Gain  Gain=j
  Mux : Mux  Inputs=2
  "Power (3ph, Instantaneous)1" : spsPower3phInstantaneousLib/Power (3ph, Instantaneous)
  Real-Imag to Complex : RealImagToComplex
  Real-Imag to Complex1 : RealImagToComplex
  Sum : Sum  Inputs=|++
  Terminator{1,3,5..8} (6 alike) : Terminator
  Transfer Fcn{1..4} (4 alike) : TransferFcn  Denominator=[1e-3 1]
  abc to Alpha-Beta-Zero : spsabctoAlphaBetaZeroLib/abc to Alpha-Beta-Zero
  abc to Alpha-Beta-Zero1 : spsabctoAlphaBetaZeroLib/abc to Alpha-Beta-Zero
  PQ : Outport
  wires:
  I/1 -> abc to Alpha-Beta-Zero1/1, "Power (3ph, Instantaneous)1"/2
  Gain1/1 -> Sum/2
  Complex to Real-Imag/1 -> Mux/1
  Complex to Real-Imag/2 -> Mux/2
  Mux/1 -> PQ/1
  "Power (3ph, Instantaneous)1"/2 -> Transfer Fcn2/1
  "Power (3ph, Instantaneous)1"/1 -> Transfer Fcn1/1
  Sum/1 -> Gain/1
  Gain/1 -> Complex to Real-Imag/1
  U/1 -> abc to Alpha-Beta-Zero/1, "Power (3ph, Instantaneous)1"/1
  abc to Alpha-Beta-Zero/1 -> Demux/1
  Demux/1 -> Real-Imag to Complex/1
  Demux/2 -> Real-Imag to Complex/2
  Real-Imag to Complex/1 -> Complex to Magnitude-Angle2/1
  Complex to Magnitude-Angle2/1 -> Transfer Fcn3/1
  Complex to Magnitude-Angle2/2 -> Terminator3/1
  Complex to Magnitude-Angle1/1 -> Transfer Fcn4/1
  Real-Imag to Complex1/1 -> Complex to Magnitude-Angle1/1
  Demux1/2 -> Real-Imag to Complex1/2
  Demux1/1 -> Real-Imag to Complex1/1
  abc to Alpha-Beta-Zero1/1 -> Demux1/1
  Transfer Fcn1/1 -> Sum/1  "p"
  Transfer Fcn2/1 -> Gain1/1  "p"
  Transfer Fcn3/1 -> Terminator6/1  "u_betrag"
  Transfer Fcn4/1 -> Terminator5/1  "i_betrag"
  Demux1/3 -> Terminator7/1
  Demux/3 -> Terminator8/1
  Complex to Magnitude-Angle1/2 -> Terminator1/1

== system power_13NodeTestFeeder_4VSC_PV_DEG_symmtrc_loads_/V I P Q Measurements EMT_without scopes_with_logsout/PQ_8 ==
  U : Inport
  I : Inport  Port=2
  Complex to Magnitude-Angle1 : ComplexToMagnitudeAngle
  Complex to Magnitude-Angle2 : ComplexToMagnitudeAngle
  Complex to Real-Imag : ComplexToRealImag
  Demux : Demux  Outputs=3
  Demux1 : Demux  Outputs=3
  Gain : Gain  Gain=1/S_base_all
  Gain1 : Gain  Gain=j
  Mux : Mux  Inputs=2
  "Power (3ph, Instantaneous)1" : spsPower3phInstantaneousLib/Power (3ph, Instantaneous)
  Real-Imag to Complex : RealImagToComplex
  Real-Imag to Complex1 : RealImagToComplex
  Sum : Sum  Inputs=|++
  Terminator{1,3,5..8} (6 alike) : Terminator
  Transfer Fcn{1..4} (4 alike) : TransferFcn  Denominator=[1e-3 1]
  abc to Alpha-Beta-Zero : spsabctoAlphaBetaZeroLib/abc to Alpha-Beta-Zero
  abc to Alpha-Beta-Zero1 : spsabctoAlphaBetaZeroLib/abc to Alpha-Beta-Zero
  PQ : Outport
  wires:
  I/1 -> abc to Alpha-Beta-Zero1/1, "Power (3ph, Instantaneous)1"/2
  Gain1/1 -> Sum/2
  Complex to Real-Imag/1 -> Mux/1
  Complex to Real-Imag/2 -> Mux/2
  Mux/1 -> PQ/1
  "Power (3ph, Instantaneous)1"/2 -> Transfer Fcn2/1
  "Power (3ph, Instantaneous)1"/1 -> Transfer Fcn1/1
  Sum/1 -> Gain/1
  Gain/1 -> Complex to Real-Imag/1
  U/1 -> abc to Alpha-Beta-Zero/1, "Power (3ph, Instantaneous)1"/1
  abc to Alpha-Beta-Zero/1 -> Demux/1
  Demux/1 -> Real-Imag to Complex/1
  Demux/2 -> Real-Imag to Complex/2
  Real-Imag to Complex/1 -> Complex to Magnitude-Angle2/1
  Complex to Magnitude-Angle2/1 -> Transfer Fcn3/1
  Complex to Magnitude-Angle2/2 -> Terminator3/1
  Complex to Magnitude-Angle1/1 -> Transfer Fcn4/1
  Real-Imag to Complex1/1 -> Complex to Magnitude-Angle1/1
  Demux1/2 -> Real-Imag to Complex1/2
  Demux1/1 -> Real-Imag to Complex1/1
  abc to Alpha-Beta-Zero1/1 -> Demux1/1
  Transfer Fcn1/1 -> Sum/1  "p"
  Transfer Fcn2/1 -> Gain1/1  "p"
  Transfer Fcn3/1 -> Terminator6/1  "u_betrag"
  Transfer Fcn4/1 -> Terminator5/1  "i_betrag"
  Demux1/3 -> Terminator7/1
  Demux/3 -> Terminator8/1
  Complex to Magnitude-Angle1/2 -> Terminator1/1

== system power_13NodeTestFeeder_4VSC_PV_DEG_symmtrc_loads_/V I P Q Measurements EMT_without scopes_with_logsout/PQ_9 ==
  U : Inport
  I : Inport  Port=2
  Complex to Magnitude-Angle1 : ComplexToMagnitudeAngle
  Complex to Magnitude-Angle2 : ComplexToMagnitudeAngle
  Complex to Real-Imag : ComplexToRealImag
  Demux : Demux  Outputs=3
  Demux1 : Demux  Outputs=3
  Gain : Gain  Gain=1/S_base_all
  Gain1 : Gain  Gain=j
  Mux : Mux  Inputs=2
  "Power (3ph, Instantaneous)1" : spsPower3phInstantaneousLib/Power (3ph, Instantaneous)
  Real-Imag to Complex : RealImagToComplex
  Real-Imag to Complex1 : RealImagToComplex
  Sum : Sum  Inputs=|++
  Terminator{1,3,5..8} (6 alike) : Terminator
  Transfer Fcn{1..4} (4 alike) : TransferFcn  Denominator=[1e-3 1]
  abc to Alpha-Beta-Zero : spsabctoAlphaBetaZeroLib/abc to Alpha-Beta-Zero
  abc to Alpha-Beta-Zero1 : spsabctoAlphaBetaZeroLib/abc to Alpha-Beta-Zero
  PQ : Outport
  wires:
  I/1 -> abc to Alpha-Beta-Zero1/1, "Power (3ph, Instantaneous)1"/2
  Gain1/1 -> Sum/2
  Complex to Real-Imag/1 -> Mux/1
  Complex to Real-Imag/2 -> Mux/2
  Mux/1 -> PQ/1
  "Power (3ph, Instantaneous)1"/2 -> Transfer Fcn2/1
  "Power (3ph, Instantaneous)1"/1 -> Transfer Fcn1/1
  Sum/1 -> Gain/1
  Gain/1 -> Complex to Real-Imag/1
  U/1 -> abc to Alpha-Beta-Zero/1, "Power (3ph, Instantaneous)1"/1
  abc to Alpha-Beta-Zero/1 -> Demux/1
  Demux/1 -> Real-Imag to Complex/1
  Demux/2 -> Real-Imag to Complex/2
  Real-Imag to Complex/1 -> Complex to Magnitude-Angle2/1
  Complex to Magnitude-Angle2/1 -> Transfer Fcn3/1
  Complex to Magnitude-Angle2/2 -> Terminator3/1
  Complex to Magnitude-Angle1/1 -> Transfer Fcn4/1
  Real-Imag to Complex1/1 -> Complex to Magnitude-Angle1/1
  Demux1/2 -> Real-Imag to Complex1/2
  Demux1/1 -> Real-Imag to Complex1/1
  abc to Alpha-Beta-Zero1/1 -> Demux1/1
  Transfer Fcn1/1 -> Sum/1  "p"
  Transfer Fcn2/1 -> Gain1/1  "p"
  Transfer Fcn3/1 -> Terminator6/1  "u_betrag"
  Transfer Fcn4/1 -> Terminator5/1  "i_betrag"
  Demux1/3 -> Terminator7/1
  Demux/3 -> Terminator8/1
  Complex to Magnitude-Angle1/2 -> Terminator1/1

== system power_13NodeTestFeeder_4VSC_PV_DEG_symmtrc_loads_/V I P Q PV_GENO_VSC Measurements/PQ_1 ==
  U : Inport
  I : Inport  Port=2
  Complex to Magnitude-Angle1 : ComplexToMagnitudeAngle
  Complex to Magnitude-Angle2 : ComplexToMagnitudeAngle
  Complex to Real-Imag : ComplexToRealImag
  Demux : Demux  Outputs=3
  Demux1 : Demux  Outputs=3
  Gain : Gain  Gain=1/S_base_all
  Gain1 : Gain  Gain=j
  Mux : Mux  Inputs=2
  "Power (3ph, Instantaneous)1" : spsPower3phInstantaneousLib/Power (3ph, Instantaneous)
  Real-Imag to Complex : RealImagToComplex
  Real-Imag to Complex1 : RealImagToComplex
  Sum : Sum  Inputs=|++
  Terminator{1,3,5..8} (6 alike) : Terminator
  Transfer Fcn{1..4} (4 alike) : TransferFcn  Denominator=[1e-3 1]
  abc to Alpha-Beta-Zero : spsabctoAlphaBetaZeroLib/abc to Alpha-Beta-Zero
  abc to Alpha-Beta-Zero1 : spsabctoAlphaBetaZeroLib/abc to Alpha-Beta-Zero
  PQ : Outport
  wires:
  I/1 -> abc to Alpha-Beta-Zero1/1, "Power (3ph, Instantaneous)1"/2
  Gain1/1 -> Sum/2
  Complex to Real-Imag/1 -> Mux/1
  Complex to Real-Imag/2 -> Mux/2
  Mux/1 -> PQ/1
  "Power (3ph, Instantaneous)1"/2 -> Transfer Fcn2/1
  "Power (3ph, Instantaneous)1"/1 -> Transfer Fcn1/1
  Sum/1 -> Gain/1
  Gain/1 -> Complex to Real-Imag/1
  U/1 -> abc to Alpha-Beta-Zero/1, "Power (3ph, Instantaneous)1"/1
  abc to Alpha-Beta-Zero/1 -> Demux/1
  Demux/1 -> Real-Imag to Complex/1
  Demux/2 -> Real-Imag to Complex/2
  Real-Imag to Complex/1 -> Complex to Magnitude-Angle2/1
  Complex to Magnitude-Angle2/1 -> Transfer Fcn3/1
  Complex to Magnitude-Angle2/2 -> Terminator3/1
  Complex to Magnitude-Angle1/1 -> Transfer Fcn4/1
  Real-Imag to Complex1/1 -> Complex to Magnitude-Angle1/1
  Demux1/2 -> Real-Imag to Complex1/2
  Demux1/1 -> Real-Imag to Complex1/1
  abc to Alpha-Beta-Zero1/1 -> Demux1/1
  Transfer Fcn1/1 -> Sum/1  "p"
  Transfer Fcn2/1 -> Gain1/1  "p"
  Transfer Fcn3/1 -> Terminator6/1  "u_betrag"
  Transfer Fcn4/1 -> Terminator5/1  "i_betrag"
  Demux1/3 -> Terminator7/1
  Demux/3 -> Terminator8/1
  Complex to Magnitude-Angle1/2 -> Terminator1/1

== system power_13NodeTestFeeder_4VSC_PV_DEG_symmtrc_loads_/V I P Q PV_GENO_VSC Measurements/PQ_2 ==
  U : Inport
  I : Inport  Port=2
  Complex to Magnitude-Angle1 : ComplexToMagnitudeAngle
  Complex to Magnitude-Angle2 : ComplexToMagnitudeAngle
  Complex to Real-Imag : ComplexToRealImag
  Demux : Demux  Outputs=3
  Demux1 : Demux  Outputs=3
  Gain : Gain  Gain=1/S_base_all
  Gain1 : Gain  Gain=j
  Mux : Mux  Inputs=2
  "Power (3ph, Instantaneous)1" : spsPower3phInstantaneousLib/Power (3ph, Instantaneous)
  Real-Imag to Complex : RealImagToComplex
  Real-Imag to Complex1 : RealImagToComplex
  Sum : Sum  Inputs=|++
  Terminator{1,3,5..8} (6 alike) : Terminator
  Transfer Fcn{1..4} (4 alike) : TransferFcn  Denominator=[1e-3 1]
  abc to Alpha-Beta-Zero : spsabctoAlphaBetaZeroLib/abc to Alpha-Beta-Zero
  abc to Alpha-Beta-Zero1 : spsabctoAlphaBetaZeroLib/abc to Alpha-Beta-Zero
  PQ : Outport
  wires:
  I/1 -> abc to Alpha-Beta-Zero1/1, "Power (3ph, Instantaneous)1"/2
  Gain1/1 -> Sum/2
  Complex to Real-Imag/1 -> Mux/1
  Complex to Real-Imag/2 -> Mux/2
  Mux/1 -> PQ/1
  "Power (3ph, Instantaneous)1"/2 -> Transfer Fcn2/1
  "Power (3ph, Instantaneous)1"/1 -> Transfer Fcn1/1
  Sum/1 -> Gain/1
  Gain/1 -> Complex to Real-Imag/1
  U/1 -> abc to Alpha-Beta-Zero/1, "Power (3ph, Instantaneous)1"/1
  abc to Alpha-Beta-Zero/1 -> Demux/1
  Demux/1 -> Real-Imag to Complex/1
  Demux/2 -> Real-Imag to Complex/2
  Real-Imag to Complex/1 -> Complex to Magnitude-Angle2/1
  Complex to Magnitude-Angle2/1 -> Transfer Fcn3/1
  Complex to Magnitude-Angle2/2 -> Terminator3/1
  Complex to Magnitude-Angle1/1 -> Transfer Fcn4/1
  Real-Imag to Complex1/1 -> Complex to Magnitude-Angle1/1
  Demux1/2 -> Real-Imag to Complex1/2
  Demux1/1 -> Real-Imag to Complex1/1
  abc to Alpha-Beta-Zero1/1 -> Demux1/1
  Transfer Fcn1/1 -> Sum/1  "p"
  Transfer Fcn2/1 -> Gain1/1  "p"
  Transfer Fcn3/1 -> Terminator6/1  "u_betrag"
  Transfer Fcn4/1 -> Terminator5/1  "i_betrag"
  Demux1/3 -> Terminator7/1
  Demux/3 -> Terminator8/1
  Complex to Magnitude-Angle1/2 -> Terminator1/1

== system power_13NodeTestFeeder_4VSC_PV_DEG_symmtrc_loads_/V I P Q PV_GENO_VSC Measurements/PQ_3 ==
  U : Inport
  I : Inport  Port=2
  Complex to Magnitude-Angle1 : ComplexToMagnitudeAngle
  Complex to Magnitude-Angle2 : ComplexToMagnitudeAngle
  Complex to Real-Imag : ComplexToRealImag
  Demux : Demux  Outputs=3
  Demux1 : Demux  Outputs=3
  Gain : Gain  Gain=1/S_base_all
  Gain1 : Gain  Gain=j
  Mux : Mux  Inputs=2
  "Power (3ph, Instantaneous)1" : spsPower3phInstantaneousLib/Power (3ph, Instantaneous)
  Real-Imag to Complex : RealImagToComplex
  Real-Imag to Complex1 : RealImagToComplex
  Sum : Sum  Inputs=|++
  Terminator{1,3,5..8} (6 alike) : Terminator
  Transfer Fcn{1..4} (4 alike) : TransferFcn  Denominator=[1e-3 1]
  abc to Alpha-Beta-Zero : spsabctoAlphaBetaZeroLib/abc to Alpha-Beta-Zero
  abc to Alpha-Beta-Zero1 : spsabctoAlphaBetaZeroLib/abc to Alpha-Beta-Zero
  PQ : Outport
  wires:
  I/1 -> abc to Alpha-Beta-Zero1/1, "Power (3ph, Instantaneous)1"/2
  Gain1/1 -> Sum/2
  Complex to Real-Imag/1 -> Mux/1
  Complex to Real-Imag/2 -> Mux/2
  Mux/1 -> PQ/1
  "Power (3ph, Instantaneous)1"/2 -> Transfer Fcn2/1
  "Power (3ph, Instantaneous)1"/1 -> Transfer Fcn1/1
  Sum/1 -> Gain/1
  Gain/1 -> Complex to Real-Imag/1
  U/1 -> abc to Alpha-Beta-Zero/1, "Power (3ph, Instantaneous)1"/1
  abc to Alpha-Beta-Zero/1 -> Demux/1
  Demux/1 -> Real-Imag to Complex/1
  Demux/2 -> Real-Imag to Complex/2
  Real-Imag to Complex/1 -> Complex to Magnitude-Angle2/1
  Complex to Magnitude-Angle2/1 -> Transfer Fcn3/1
  Complex to Magnitude-Angle2/2 -> Terminator3/1
  Complex to Magnitude-Angle1/1 -> Transfer Fcn4/1
  Real-Imag to Complex1/1 -> Complex to Magnitude-Angle1/1
  Demux1/2 -> Real-Imag to Complex1/2
  Demux1/1 -> Real-Imag to Complex1/1
  abc to Alpha-Beta-Zero1/1 -> Demux1/1
  Transfer Fcn1/1 -> Sum/1  "p"
  Transfer Fcn2/1 -> Gain1/1  "p"
  Transfer Fcn3/1 -> Terminator6/1  "u_betrag"
  Transfer Fcn4/1 -> Terminator5/1  "i_betrag"
  Demux1/3 -> Terminator7/1
  Demux/3 -> Terminator8/1
  Complex to Magnitude-Angle1/2 -> Terminator1/1

== system power_13NodeTestFeeder_4VSC_PV_DEG_symmtrc_loads_/V I P Q PV_GENO_VSC Measurements/PQ_4 ==
  U : Inport
  I : Inport  Port=2
  Complex to Magnitude-Angle1 : ComplexToMagnitudeAngle
  Complex to Magnitude-Angle2 : ComplexToMagnitudeAngle
  Complex to Real-Imag : ComplexToRealImag
  Demux : Demux  Outputs=3
  Demux1 : Demux  Outputs=3
  Gain : Gain  Gain=1/S_base_all
  Gain1 : Gain  Gain=j
  Mux : Mux  Inputs=2
  "Power (3ph, Instantaneous)1" : spsPower3phInstantaneousLib/Power (3ph, Instantaneous)
  Real-Imag to Complex : RealImagToComplex
  Real-Imag to Complex1 : RealImagToComplex
  Sum : Sum  Inputs=|++
  Terminator{1,3,5..8} (6 alike) : Terminator
  Transfer Fcn{1..4} (4 alike) : TransferFcn  Denominator=[1e-3 1]
  abc to Alpha-Beta-Zero : spsabctoAlphaBetaZeroLib/abc to Alpha-Beta-Zero
  abc to Alpha-Beta-Zero1 : spsabctoAlphaBetaZeroLib/abc to Alpha-Beta-Zero
  PQ : Outport
  wires:
  I/1 -> abc to Alpha-Beta-Zero1/1, "Power (3ph, Instantaneous)1"/2
  Gain1/1 -> Sum/2
  Complex to Real-Imag/1 -> Mux/1
  Complex to Real-Imag/2 -> Mux/2
  Mux/1 -> PQ/1
  "Power (3ph, Instantaneous)1"/2 -> Transfer Fcn2/1
  "Power (3ph, Instantaneous)1"/1 -> Transfer Fcn1/1
  Sum/1 -> Gain/1
  Gain/1 -> Complex to Real-Imag/1
  U/1 -> abc to Alpha-Beta-Zero/1, "Power (3ph, Instantaneous)1"/1
  abc to Alpha-Beta-Zero/1 -> Demux/1
  Demux/1 -> Real-Imag to Complex/1
  Demux/2 -> Real-Imag to Complex/2
  Real-Imag to Complex/1 -> Complex to Magnitude-Angle2/1
  Complex to Magnitude-Angle2/1 -> Transfer Fcn3/1
  Complex to Magnitude-Angle2/2 -> Terminator3/1
  Complex to Magnitude-Angle1/1 -> Transfer Fcn4/1
  Real-Imag to Complex1/1 -> Complex to Magnitude-Angle1/1
  Demux1/2 -> Real-Imag to Complex1/2
  Demux1/1 -> Real-Imag to Complex1/1
  abc to Alpha-Beta-Zero1/1 -> Demux1/1
  Transfer Fcn1/1 -> Sum/1  "p"
  Transfer Fcn2/1 -> Gain1/1  "p"
  Transfer Fcn3/1 -> Terminator6/1  "u_betrag"
  Transfer Fcn4/1 -> Terminator5/1  "i_betrag"
  Demux1/3 -> Terminator7/1
  Demux/3 -> Terminator8/1
  Complex to Magnitude-Angle1/2 -> Terminator1/1

== system power_13NodeTestFeeder_4VSC_PV_DEG_symmtrc_loads_/PV_Geno_GFL_VSC_at_634/PV-Geno with VSC_GFL_at_634     /PV Array ==
  note: Allows PV model to initialize
  T : Inport
  G : Inport  Port=2
  V_dc : Inport  Port=3
  I_dc : Inport  Port=4
  Controlled Current Source19 : spsControlledCurrentSourceLib/Controlled Current Source  Initialize=on  Source_Type=AC  Amplitude=0  Phase=0  Frequency=0  Measurements=None
  Display : Display
  I module : MATLABFcn  MATLABFcn=Np*u(2)-Np*u(1)*(exp((u(3)/(Ns)+Rs*u(4)/Np)/((Ns_cell*k*(u(5)+273.15)/q)*a))-1)-Np*((u(3)/(Ns)+Rs*u(4)/Np)/Rp)  OutputDimensions=1
  I0 : MATLABFcn  MATLABFcn=(Isc_n+KI*(u(1)-Tn))/(exp((Voc_n+KV*(u(1)-Tn))/((Ns_cell*k*(u(1)+273.15)/q)*a))-1);  OutputDimensions=1
  Ipv : MATLABFcn  MATLABFcn=(Ipv_n+KI*(u(1)-Tn))*(u(2)/Gn);  OutputDimensions=1
  Memory : Memory
  Memory1 : Memory
  Mux : Mux  Inputs=2
  Mux1 : Mux  Inputs=5
  Product17 : Product
  Saturation : Saturate  UpperLimit=10e6  LowerLimit=0.1
  Step16 : Step  Time=0.001  SampleTime=0
  PV+ : PMIOPort  Side=Right
  PV- : PMIOPort  Port=2  Side=Right
  wires:
  Mux1/1 -> I module/1
  G/1 -> Mux/2
  Mux/1 -> Ipv/1
  T/1 -> Mux1/5, Mux/1, I0/1
  Ipv/1 -> Mux1/2
  I0/1 -> Mux1/1
  Memory/1 -> Mux1/4
  I_dc/1 -> Memory/1
  Saturation/1 -> Product17/1
  Step16/1 -> Product17/2
  Product17/1 -> Controlled Current Source19/1
  Memory1/1 -> Mux1/3
  V_dc/1 -> Memory1/1
  I module/1 -> Display/1, Saturation/1
  connections:
  PV+/RConn1 -- Controlled Current Source19/RConn1
  Controlled Current Source19/LConn1 -- PV-/RConn1

== system power_13NodeTestFeeder_4VSC_PV_DEG_symmtrc_loads_/PV_Geno_GFL_VSC_at_634/PV-Geno with VSC_GFL_at_634     /VSC ==
  V_abc_c : Inport
  I_abc_c : Inport  Port=2
  V_dc : Inport  Port=3
  Controlled Current Source1 : spsControlledCurrentSourceLib/Controlled Current Source  Initialize=on  Source_Type=AC  Amplitude=0  Phase=0  Frequency=0  Measurements=None
  Controlled Voltage Source3 : spsControlledVoltageSourceLib/Controlled Voltage Source  Initialize=off  Source_Type=AC  Amplitude=0  Phase=0  Frequency=60  Measurements=None
  Controlled Voltage Source4 : spsControlledVoltageSourceLib/Controlled Voltage Source  Initialize=off  Source_Type=AC  Amplitude=0  Phase=0  Frequency=60  Measurements=None
  Controlled Voltage Source5 : spsControlledVoltageSourceLib/Controlled Voltage Source  Initialize=off  Source_Type=AC  Amplitude=0  Phase=0  Frequency=60  Measurements=None
  Delay : Delay  DelayLength=1  InitialCondition=1200
  Demux : Demux  Outputs=3
  Divide : Product  Inputs=*/  RndMeth=Zero  SaturateOnIntegerOverflow=on
  Ground : spsGroundLib/Ground  LConnTagsString=a
  Product : Product
  Sum of Elements : Sum  Inputs=+
  Va_c : PMIOPort  Side=Left
  Vb_c : PMIOPort  Port=2  Side=Left
  Vc_c : PMIOPort  Port=3  Side=Left
  dc+ : PMIOPort  Port=4  Side=Right
  dc- : PMIOPort  Port=5  Side=Right
  wires:
  Product/1 -> Sum of Elements/1
  I_abc_c/1 -> Product/2
  V_abc_c/1 -> Demux/1, Product/1
  Demux/2 -> Controlled Voltage Source4/1
  Demux/1 -> Controlled Voltage Source3/1
  Demux/3 -> Controlled Voltage Source5/1
  Sum of Elements/1 -> Divide/1
  Divide/1 -> Controlled Current Source1/1
  V_dc/1 -> Delay/1
  Delay/1 -> Divide/2
  connections:
  Vb_c/RConn1 -- Controlled Voltage Source4/RConn1
  Va_c/RConn1 -- Controlled Voltage Source3/RConn1
  Controlled Voltage Source4/LConn1 -- Controlled Voltage Source3/LConn1 -- Controlled Voltage Source5/LConn1 -- Ground/LConn1
  Vc_c/RConn1 -- Controlled Voltage Source5/RConn1
  Controlled Current Source1/RConn1 -- dc-/RConn1
  dc+/RConn1 -- Controlled Current Source1/LConn1
